simulink model "DriveSimulation"  (R2019b)
settings: Solver=FixedStepAuto  StartTime=0.0  StopTime=inf  FixedStep=dt  RelTol=1e-3
model workspace (MAT data in the model file):
  AcceNoisePower = 0.01
  AcceNoiseStd = 0.1
  AcceTs = 0.01
  ControlTs = 0.1
  DeltaNoiseStd = 0.000174532925199
  GPSNoisePower = 0.001
  GPSNoiseStd = 1
  GPSTs = 0.5
  GyroNoisePower = 0.001
  GyroNoiseStd = 0.000174532925199
  GyroTs = 0.01
  L = 2
  SteeringRange = 0.837758040957
  Ts = 0.01
  Var = 0
  Vmax = 41.6666666667
  dt = 0.01
undefined symbols (not defined in the file): DiscIntNeverNeededParam
libraries: simulink x2, robotmobilelib x1, sim3dlib x1, sim3dautolib x1, aerolibanimutils x1
settings Model: Creator=alons  LastModifiedBy=alons
settings DataIOCC: ReturnWorkspaceOutputs=off
settings DebuggingCC: ArithmeticOperatorsInVariantConditions=warning
settings SFSimCC: CustomCodeUndefinedFunction=UseInterfaceOnly

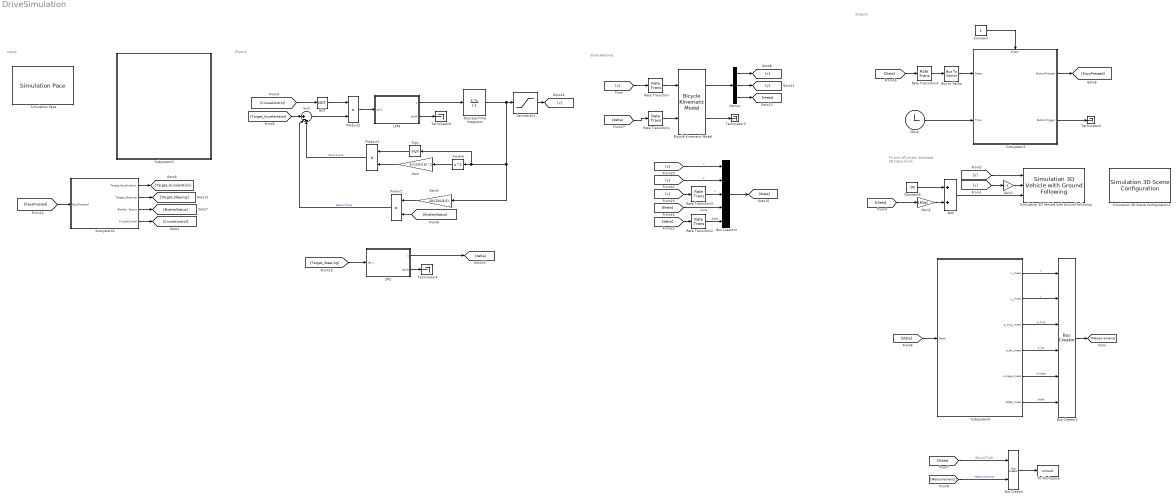
== system DriveSimulation ==
  note: Physics
  note: State Advance
  note: Inputs
  note: Outputs
  note: To turn off unreal:
      | Annotate 3D scene block
  Add : Sum
  Bicycle Kinematic Model : robotmobilelib/Bicycle Kinematic Model  VehicleInputs=Vehicle Speed & Steering Angle  WheelBase=L  VehicleSpeedRange=[-Vmax/3 Vmax]  MaxSteeringAngle=SteeringRange/2  InitialState=[0; 0; pi/2]  SimulateUsing=Interpreted execution
      settings: SourceProductName=Robotics System Toolbox  SourceProductBaseCode=RO
  Bus Creator : BusCreator  Inputs=2
  Bus Creator2 : BusCreator  Inputs=6
  Bus Creator3 : BusCreator  Inputs=5
  Bus to Vector : BusToVector
  Clock : Clock
  Constant : Constant  SampleTime=0
      settings: OpenFcn=|
      | if get_param(gcbh,'value')-48
      |    set_param(gcbh,'value','0','backgroundcolor','red');
      | else
      |    set_param(gcbh,'value','1','backgroundcolor','green');
      | end
  Constant6 : Constant  Value=-90
  Demux : Demux  Outputs=3
  Discrete-Time Integrator : DiscreteIntegrator  SampleTime=-1  ICPrevOutput=DiscIntNeverNeededParam  ICPrevScaledInput=DiscIntNeverNeededParam
  Gain : Gain  Gain=5/(150/3.6)^2
  Gain1 : Gain  Gain=-1
  Gain2 : Gain  Gain=180/pi
  Gain3 : Gain  Gain=20/(150/3.6)
  LPF2 : Subsystem  mask{Freq=2}
      mask prompts: Freq "LPF Freq [Hz]"
      mask Display: fprintf('LPF %g[Hz]',Freq);
  LPF3 : Subsystem  mask{Freq=2}
      mask prompts: Freq "LPF Freq [Hz]"
      mask Display: fprintf('LPF %g[Hz]',Freq);
  NOT : Logic  Operator=NOT  AllPortsSameDT=off  OutDataTypeStr=boolean
  Product : Product
  Product1 : Product
  Product2 : Product
  Rate Transition{,1..3} (4 alike) : RateTransition  OutPortSampleTime=dt
  Rate Transition4 : RateTransition  OutPortSampleTime=ControlTs
  Saturation1 : Saturate  UpperLimit=Vmax  LowerLimit=-Vmax/3
  Sign : Signum
  Simulation 3D Scene Configuration1 : sim3dlib/Simulation 3D Scene Configuration  Priority=0  SceneDesc=Curved road  vehTagList={'Scene Origin';'SimulinkVehicle1'}  vehTag=SimulinkVehicle1  OpVisEn=off  Ts=ControlTs  ProjectFormat=Executable  ProjectName=VehicleSimulation.exe  sensorTag=MainCamera1  sensorId=1  sensorName=MainCamera1  mountLoc=Origin  offsetFlag=off  tmountOffset=[0, 0, 0]  rmountOffset=[0, 0, 0]  HorizontalResolution=1280  VerticalResolution=720  HorizontalFOV=60  mountPoint=[0 0 0]  mountOrientation=[0 0 0]  aMode=3  ID=1
      settings: SourceProductName=Automated Driving Toolbox  SourceProductBaseCode=DR
  Simulation 3D Vehicle with Ground Following : sim3dautolib/Simulation 3D Vehicle with Ground Following  Priority=-1  PassVehMesh=Muscle car  VehColor=Red  InitialPos=[0, 0, 0]  InitialRot=[0, 0, 0]  ActorName=SimulinkVehicle1  SampleTime=-1  ActorType=SimulinkVehicle  ID=1  aMode=3  ActorTag=SimulinkVehicle1  CoordinateScheme=ISO  TransformOutportEnabled=off
      settings: SourceProductName=Automated Driving Toolbox  SourceProductBaseCode=DR
  Simulation Pace : aerolibanimutils/Simulation Pace  SimulationPace=1  SleepMode=Auto  OutputPaceError=off  SampleTime=dt
  Square : Math  Operator=square  SignedPower=off  SaturateOnIntegerOverflow=on
  Subsystem1 : Subsystem  InitFcn=|  mask{dt=0.01, ControlTs=0.1, AcceTs=0.01, GyroTs=0.01, GPSTs=0.5, AcceNoiseStd=0.1, GyroNoiseStd=0.01*pi/180, GPSNoiseStd=1, DeltaNoiseStd=0.01/180*pi, L=2, Vmax=150/3.6, SteeringRange=48/180*pi}
      | mdlWks=get_param(bdroot,'ModelWorkspace')
      | par = get_param(gcb,'DialogParameters');
      | fnames = fieldnames(par);
      | for ipar=1:length(fnames)
      |    num=str2num(get_param(gcb,fnames{ipar}));
      |    mdlWks.assignin(fnames{ipar},num);
      | end
      | 
      | clear par fnames ipar num mdlWks;
      mask prompts: dt "Physics Time Sample [s]"; ControlTs "Control Time Sample [s]"; AcceTs "Accelerometer Time Sample [s]"; GyroTs "Gyro Time Sample [s]"; GPSTs "GPS Time Sample [s]"; AcceNoiseStd "Accelerometer Noise std [m/s^2]"; GyroNoiseStd "Gyro Noise std [rad/s]"; GPSNoiseStd "GPS Noise std [m]"; DeltaNoiseStd "Steering Wheel Noise std [rad]"; L "Bicycle Length [m]"; Vmax "Maximum Velocity [m/s]"; SteeringRange "Steering Range [rad]"
      mask Display:
      | str=[
      |     'Model Workspace Parameters \n\n\n',...
      |     'Physics Sample dt = %g[s]\n\n',...
      |     'Control Sample ControlTs = %g[s]\n\n',...
      |     'Accelerometer Sample AcceTs = %g[s]\n\n',...
      |     'Gyro Sample GyroTs = %g[s]\n\n',...
      |     'GPS Sample GpsTs = %g[s]\n\n',...
      |     'Accelerometer Noise std = %g[m/s^2]\n\n',...
      |     'Gyro Noise std = %g[rad/s^2]\n\n',...
      |     'GPS Noise std = %g[m]\n\n',...
      |     'Steering Wheel Noise std = %g[m]\n\n',...
      |     'Bicycle Length L = %g[m]\n\n',...
      |     'Maximum Velocity Vmax = %g[m/s]\n\n',...
      |     'SteeringRange = %g[rad]\n\n',...
      |     ];
      | fprintf(str,dt,ControlTs,AcceTs,GyroTs,GPSTs,...
      |     AcceNoiseStd,GyroNoiseStd,GPSNoiseStd,DeltaNoiseStd,L,Vmax,SteeringRange);
  Subsystem2 : Subsystem
      settings: OpenFcn=|
      | UserData = get_param([gcb,'/AnimationSfcn'],'UserData');
      | Fig = UserData.Figure;
      | if ishghandle(Fig,'figure');
      |    %bring to the front:
      |    figure(Fig);
      | end
      mask Display:
      | t=linspace(0,2*pi,20);
      | plot(cos(t),sin(t));
      | 
      | x=[-0.4,-0.4,0.6,-0.4];
      | y=[-0.5,0.5,0,-0.5];
      | plot(x,y)
      | 
      | disp('Drive Simulator')
  Subsystem3 : Subsystem
  Subsystem4 : Subsystem
      mask Display: disp('Sensor Readings')
  Sum : Sum  Inputs=||+--
  Terminator{2..5} (4 alike) : Terminator
  To Workspace : ToWorkspace  VariableName=simout  SaveFormat=Timeseries  SampleTime=-1
  wires:
  Constant/1 -> Subsystem2/Enable
  Clock/1 -> Subsystem2/2(Time)
  Subsystem3/1(Target_Acceleration) -> [Target_Acceleration]
  Subsystem3/2(Target_Steering) -> [Target_Steering]
  Bus to Vector/1 -> Subsystem2/1(State)
  Subsystem2/1(ButtonPressed) -> [KeysPressed]
  Subsystem2/2(ButtonTrigger) -> Terminator2/1
  Subsystem4/5(omega_meas) -> Bus Creator2/5  "omega"
  Subsystem4/4(a_lat_meas) -> Bus Creator2/4  "a_lat"
  Subsystem4/3(a_long_meas) -> Bus Creator2/3  "a_long"
  Subsystem4/2(y_meas) -> Bus Creator2/2  "y"
  Subsystem4/1(x_meas) -> Bus Creator2/1  "x"
  Subsystem4/6(delta_meas) -> Bus Creator2/6  "delta"
  [KeysPressed] -> Subsystem3/1(KeysPressed)
  Bicycle Kinematic Model/2 -> Terminator3/1
  Bicycle Kinematic Model/1 -> Demux/1
  Demux/1 -> [x]
  Demux/2 -> [y]
  Demux/3 -> [theta]
  [x] -> Bus Creator3/1  "x"
  [y] -> Bus Creator3/2  "y"
  [v] -> Rate Transition3/1
  [theta] -> Bus Creator3/4  "theta"
  [delta] -> Rate Transition2/1
  Bus Creator3/1 -> [State]
  [State] -> Rate Transition4/1
  [Target_Steering] -> LPF2/1(ref s)
  LPF2/1(s) -> [delta]
  LPF2/2(ds/dt) -> Terminator4/1
  [delta] -> Rate Transition1/1
  [v] -> Rate Transition/1
  [State] -> Subsystem4/1(State)
  LPF3/1(s) -> Discrete-Time Integrator/1
  LPF3/2(ds/dt) -> Terminator5/1
  [Target_Acceleration] -> Sum/1
  Square/1 -> Gain/1
  Discrete-Time Integrator/1 -> Gain3/1, Sign/1, Square/1, Saturation1/1
  Subsystem3/3(Brakes  Status) -> [BrakesStatus]
  Gain3/1 -> Product/1
  Product/1 -> Sum/2  "Brake Force"
  [BrakesStatus] -> Product/2
  [theta] -> Gain2/1
  [y] -> Simulation 3D Vehicle with Ground Following/1
  Constant6/1 -> Add/1
  Gain2/1 -> Add/2
  Add/1 -> Simulation 3D Vehicle with Ground Following/3
  [x] -> Gain1/1
  Gain1/1 -> Simulation 3D Vehicle with Ground Following/2
  Product1/1 -> Sum/3  "Wind Force"
  Gain/1 -> Product1/2
  Sign/1 -> Product1/1
  Bus Creator2/1 -> [Measurements]
  Bus Creator/1 -> To Workspace/1
  [State] -> Bus Creator/1  "Ground Truth"
  [Measurements] -> Bus Creator/2  "Measurements"
  Subsystem3/4(CruiseControl) -> [CruiseControl]
  Sum/1 -> Product2/2
  [CruiseControl] -> NOT/1
  NOT/1 -> Product2/1
  Product2/1 -> LPF3/1(ref s)
  Saturation1/1 -> [v]
  Rate Transition/1 -> Bicycle Kinematic Model/1
  Rate Transition1/1 -> Bicycle Kinematic Model/2
  Rate Transition2/1 -> Bus Creator3/5  "delta"
  Rate Transition3/1 -> Bus Creator3/3  "v"
  Rate Transition4/1 -> Bus to Vector/1

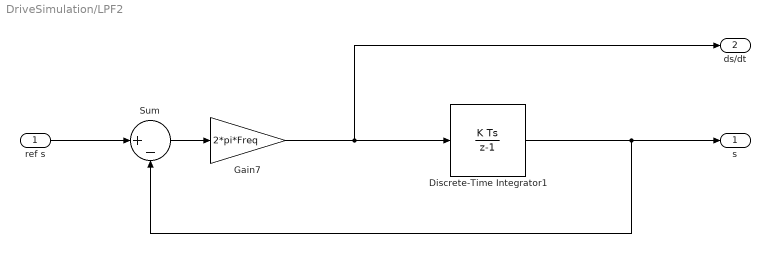
== system DriveSimulation/LPF2 ==
  ref s : Inport
  Discrete-Time Integrator1 : DiscreteIntegrator  SampleTime=-1  ICPrevOutput=DiscIntNeverNeededParam  ICPrevScaledInput=DiscIntNeverNeededParam
  Gain7 : Gain  Gain=2*pi*Freq
  Sum : Sum  Inputs=|+-
  s : Outport  VectorParamsAs1DForOutWhenUnconnected=off
  ds/dt : Outport  Port=2  VectorParamsAs1DForOutWhenUnconnected=off
  wires:
  Discrete-Time Integrator1/1 -> Sum/2, s/1
  Sum/1 -> Gain7/1
  ref s/1 -> Sum/1
  Gain7/1 -> Discrete-Time Integrator1/1, ds/dt/1

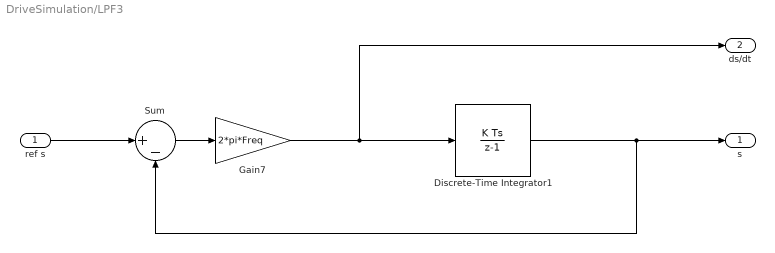
== system DriveSimulation/LPF3 ==
  ref s : Inport
  Discrete-Time Integrator1 : DiscreteIntegrator  SampleTime=-1  ICPrevOutput=DiscIntNeverNeededParam  ICPrevScaledInput=DiscIntNeverNeededParam
  Gain7 : Gain  Gain=2*pi*Freq
  Sum : Sum  Inputs=|+-
  s : Outport  VectorParamsAs1DForOutWhenUnconnected=off
  ds/dt : Outport  Port=2  VectorParamsAs1DForOutWhenUnconnected=off
  wires:
  Discrete-Time Integrator1/1 -> Sum/2, s/1
  Sum/1 -> Gain7/1
  ref s/1 -> Sum/1
  Gain7/1 -> Discrete-Time Integrator1/1, ds/dt/1

== system DriveSimulation/Subsystem1 ==

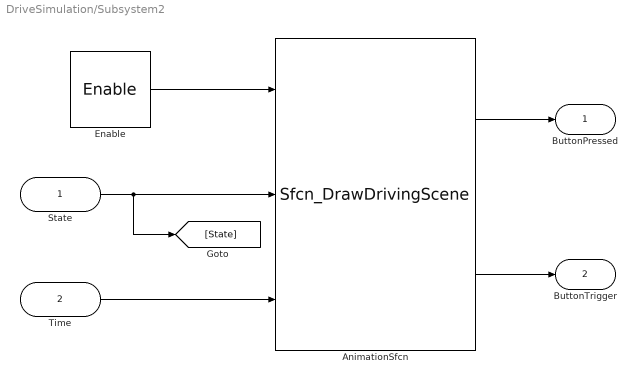
== system DriveSimulation/Subsystem2 ==
  State : Inport
  Time : Inport  Port=2
  Enable : EnablePort  StatesWhenEnabling=reset  ShowOutputPort=on
  AnimationSfcn : M-S-Function  FunctionName=Sfcn_DrawDrivingScene  Parameters=ControlTs,L,Vmax
  ButtonPressed : Outport  VectorParamsAs1DForOutWhenUnconnected=off
  ButtonTrigger : Outport  Port=2  VectorParamsAs1DForOutWhenUnconnected=off
  wires:
  Enable/1 -> AnimationSfcn/1
  AnimationSfcn/1 -> ButtonPressed/1
  AnimationSfcn/2 -> ButtonTrigger/1
  Time/1 -> AnimationSfcn/3
  State/1 -> [State], AnimationSfcn/2

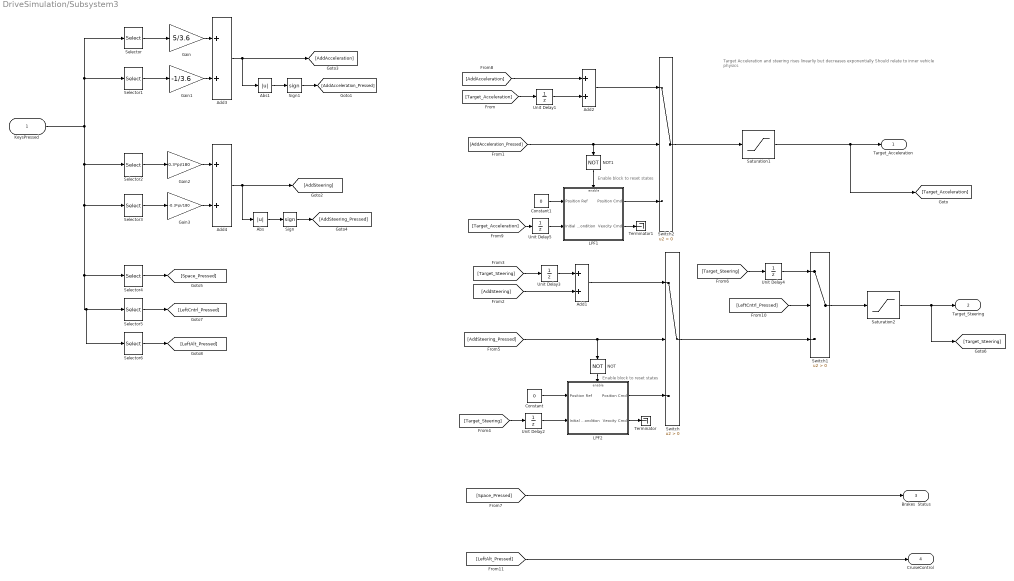
== system DriveSimulation/Subsystem3 ==
  note: Enable block to reset states
  note: Enable block to reset states
  note: Target Acceleration and steering rises linearliy but decreases exponentially
      | Should relate to inner vehicle physics
  KeysPressed : Inport
  Abs : Abs
  Abs1 : Abs
  Add{1..4} (4 alike) : Sum
  Constant : Constant  Value=0
  Constant1 : Constant  Value=0
  Gain : Gain  Gain=5/3.6
  Gain1 : Gain  Gain=-1/3.6
  Gain2 : Gain  Gain=0.3*pi/180
  Gain3 : Gain  Gain=-0.3*pi/180
  LPF1 : Subsystem  mask{PosBW=1, Vel_Max=inf, Vel_Min=-inf}
      mask prompts: PosBW "Position BW [Hz]"; Vel_Max "Maximum Velocity"; Vel_Min "Minimum Velocity"
      mask Display: fprintf('Resetable LPF %.3g[Hz] \n/w Vel Limits',PosBW);
  LPF2 : Subsystem  mask{PosBW=0.5, Vel_Max=inf, Vel_Min=-inf}
      mask prompts: PosBW "Position BW [Hz]"; Vel_Max "Maximum Velocity"; Vel_Min "Minimum Velocity"
      mask Display: fprintf('Resetable LPF %.3g[Hz] \n/w Vel Limits',PosBW);
  NOT : Logic  Operator=NOT  AllPortsSameDT=off  OutDataTypeStr=boolean
  NOT1 : Logic  Operator=NOT  AllPortsSameDT=off  OutDataTypeStr=boolean
  Saturation1 : Saturate  UpperLimit=10  LowerLimit=-10
  Saturation2 : Saturate  UpperLimit=SteeringRange/2  LowerLimit=-SteeringRange/2
  Selector : Selector  InputPortWidth=7  IndexOptions=Index vector (dialog)  Indices=1  OutputSizes=1
  Selector1 : Selector  InputPortWidth=7  IndexOptions=Index vector (dialog)  Indices=2  OutputSizes=1
  Selector2 : Selector  InputPortWidth=7  IndexOptions=Index vector (dialog)  Indices=3  OutputSizes=1
  Selector3 : Selector  InputPortWidth=7  IndexOptions=Index vector (dialog)  Indices=4  OutputSizes=1
  Selector4 : Selector  InputPortWidth=7  IndexOptions=Index vector (dialog)  Indices=5  OutputSizes=1
  Selector5 : Selector  InputPortWidth=7  IndexOptions=Index vector (dialog)  Indices=6  OutputSizes=1
  Selector6 : Selector  InputPortWidth=7  IndexOptions=Index vector (dialog)  Indices=7  OutputSizes=1
  Sign : Signum
  Sign1 : Signum
  Switch : Switch  Criteria=u2 > Threshold
  Switch1 : Switch  Criteria=u2 > Threshold
  Switch2 : Switch  Criteria=u2 > Threshold
  Terminator : Terminator
  Terminator1 : Terminator
  Unit Delay{1..5} (5 alike) : UnitDelay  SampleTime=-1  HasFrameUpgradeWarning=on
  Target_Acceleration : Outport  VectorParamsAs1DForOutWhenUnconnected=off
  Target_Steering : Outport  Port=2  VectorParamsAs1DForOutWhenUnconnected=off
  Brakes  Status : Outport  Port=3  VectorParamsAs1DForOutWhenUnconnected=off
  CruiseControl : Outport  Port=4  VectorParamsAs1DForOutWhenUnconnected=off
  wires:
  [Target_Acceleration] -> Unit Delay1/1
  Unit Delay1/1 -> Add2/2
  Add2/1 -> Switch2/1
  [AddAcceleration] -> Add2/1
  Add4/1 -> Abs/1, [AddSteering]
  Selector/1 -> Gain/1
  Selector1/1 -> Gain1/1
  Gain1/1 -> Add3/2
  Gain/1 -> Add3/1
  Add3/1 -> Abs1/1, [AddAcceleration]
  Selector2/1 -> Gain2/1
  Selector3/1 -> Gain3/1
  Gain2/1 -> Add4/1
  Gain3/1 -> Add4/2
  Switch2/1 -> Saturation1/1
  KeysPressed/1 -> Selector6/1, Selector5/1, Selector4/1, Selector3/1, Selector2/1, Selector/1, Selector1/1
  Abs/1 -> Sign/1
  Sign/1 -> [AddSteering_Pressed]
  Selector4/1 -> [Space_Pressed]
  Switch1/1 -> Saturation2/1
  Unit Delay2/1 -> LPF2/2(Initial Condition)
  [Target_Steering] -> Unit Delay3/1
  [Target_Steering] -> Unit Delay2/1
  LPF2/2(Veocity Cmd) -> Terminator/1
  Unit Delay3/1 -> Add1/1
  [AddSteering] -> Add1/2
  LPF2/1(Position Cmd) -> Switch/3
  Constant/1 -> LPF2/1(Position Ref)
  NOT/1 -> LPF2/Enable
  [AddSteering_Pressed] -> NOT/1, Switch/2
  Add1/1 -> Switch/1
  [LeftCntrl_Pressed] -> Switch1/2
  [Target_Steering] -> Unit Delay4/1
  Unit Delay4/1 -> Switch1/1
  Switch/1 -> Switch1/3
  Abs1/1 -> Sign1/1
  Sign1/1 -> [AddAcceleration_Pressed]
  Unit Delay5/1 -> LPF1/2(Initial Condition)
  LPF1/1(Position Cmd) -> Switch2/3
  LPF1/2(Veocity Cmd) -> Terminator1/1
  Constant1/1 -> LPF1/1(Position Ref)
  [AddAcceleration_Pressed] -> Switch2/2, NOT1/1
  NOT1/1 -> LPF1/Enable
  [Target_Acceleration] -> Unit Delay5/1
  Saturation1/1 -> Target_Acceleration/1, [Target_Acceleration]
  Saturation2/1 -> [Target_Steering], Target_Steering/1
  Selector5/1 -> [LeftCntrl_Pressed]
  [Space_Pressed] -> Brakes  Status/1
  Selector6/1 -> [LeftAlt_Pressed]
  [LeftAlt_Pressed] -> CruiseControl/1

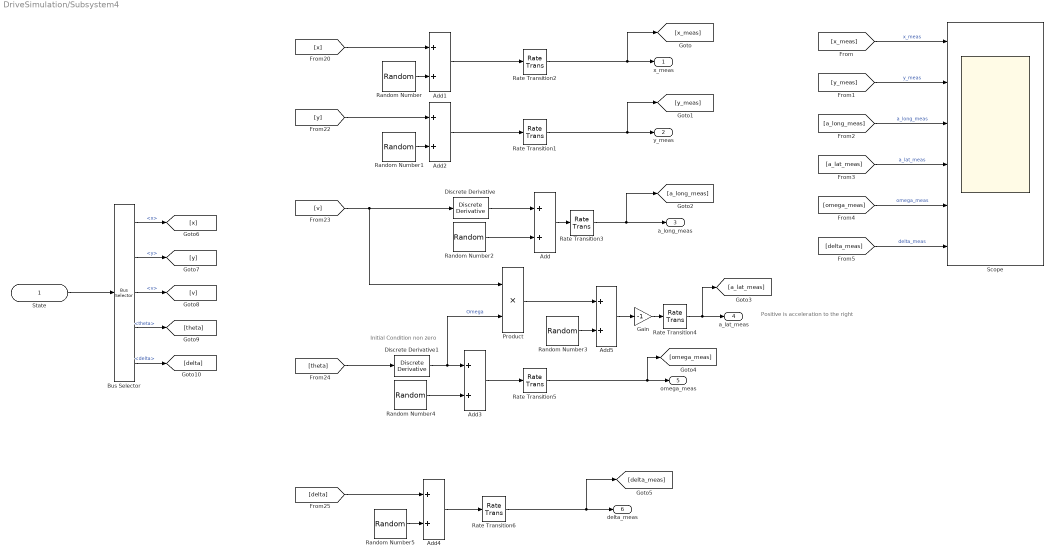
== system DriveSimulation/Subsystem4 ==
  note: Initial Condition non zero
  note: Positive is acceleration to the right
  State : Inport
  Add{,1..5} (6 alike) : Sum
  Bus Selector : BusSelector  OutputSignals=x,y,v,theta,delta
  Discrete Derivative : simulink/Discrete/Discrete Derivative  gainval=1.0  ICPrevScaledInput=0.0  OutMin=[]  OutMax=[]  OutDataType=fixdt(1, 16)  OutScaling=2^-10  DoSatur=off
  Discrete Derivative1 : simulink/Discrete/Discrete Derivative  gainval=1.0  ICPrevScaledInput=pi/2/dt  OutMin=[]  OutMax=[]  OutDataType=fixdt(1, 16)  OutScaling=2^-10  DoSatur=off
  Gain : Gain  Gain=-1
  Product : Product
  Random Number : RandomNumber  Variance=(GPSNoiseStd^2)
  Random Number1 : RandomNumber  Variance=(GPSNoiseStd^2)  Seed=2
  Random Number2 : RandomNumber  Variance=AcceNoiseStd^2  Seed=3
  Random Number3 : RandomNumber  Variance=AcceNoiseStd^2  Seed=4
  Random Number4 : RandomNumber  Variance=GyroNoiseStd  Seed=5
  Random Number5 : RandomNumber  Variance=(DeltaNoiseStd^2)  Seed=2
  Rate Transition1 : RateTransition  OutPortSampleTime=GPSTs
  Rate Transition2 : RateTransition  OutPortSampleTime=GPSTs
  Rate Transition3 : RateTransition  OutPortSampleTime=AcceTs
  Rate Transition4 : RateTransition  OutPortSampleTime=AcceTs
  Rate Transition5 : RateTransition  OutPortSampleTime=GyroTs
  Rate Transition6 : RateTransition  OutPortSampleTime=GPSTs
  Scope : Scope  NumInputPorts=6
  x_meas : Outport  VectorParamsAs1DForOutWhenUnconnected=off
  y_meas : Outport  Port=2  VectorParamsAs1DForOutWhenUnconnected=off
  a_long_meas : Outport  Port=3  VectorParamsAs1DForOutWhenUnconnected=off
  a_lat_meas : Outport  Port=4  VectorParamsAs1DForOutWhenUnconnected=off
  omega_meas : Outport  Port=5  VectorParamsAs1DForOutWhenUnconnected=off
  delta_meas : Outport  Port=6  VectorParamsAs1DForOutWhenUnconnected=off
  wires:
  Random Number/1 -> Add1/2
  Random Number2/1 -> Add/2
  Random Number3/1 -> Add5/2
  Random Number1/1 -> Add2/2
  [v] -> Product/1, Discrete Derivative/1
  Discrete Derivative1/1 -> Product/2, Add3/1  "Omega"
  Product/1 -> Add5/1
  [y] -> Add2/1
  Random Number4/1 -> Add3/2
  Add1/1 -> Rate Transition2/1
  Add/1 -> Rate Transition3/1
  Add3/1 -> Rate Transition5/1
  Add2/1 -> Rate Transition1/1
  [x] -> Add1/1
  Add5/1 -> Gain/1
  [theta] -> Discrete Derivative1/1
  Gain/1 -> Rate Transition4/1
  [x_meas] -> Scope/1  "x_meas"
  [y_meas] -> Scope/2  "y_meas"
  [a_long_meas] -> Scope/3  "a_long_meas"
  [a_lat_meas] -> Scope/4  "a_lat_meas"
  [omega_meas] -> Scope/5  "omega_meas"
  Rate Transition2/1 -> [x_meas], x_meas/1
  Rate Transition1/1 -> [y_meas], y_meas/1
  Rate Transition3/1 -> [a_long_meas], a_long_meas/1
  Rate Transition4/1 -> [a_lat_meas], a_lat_meas/1
  Rate Transition5/1 -> [omega_meas], omega_meas/1
  Discrete Derivative/1 -> Add/1
  [delta] -> Add4/1
  Rate Transition6/1 -> [delta_meas], delta_meas/1
  Add4/1 -> Rate Transition6/1
  Random Number5/1 -> Add4/2
  [delta_meas] -> Scope/6  "delta_meas"
  State/1 -> Bus Selector/1
  Bus Selector/1 -> [x]  "<x>"
  Bus Selector/2 -> [y]  "<y>"
  Bus Selector/3 -> [v]  "<v>"
  Bus Selector/4 -> [theta]  "<theta>"
  Bus Selector/5 -> [delta]  "<delta>"

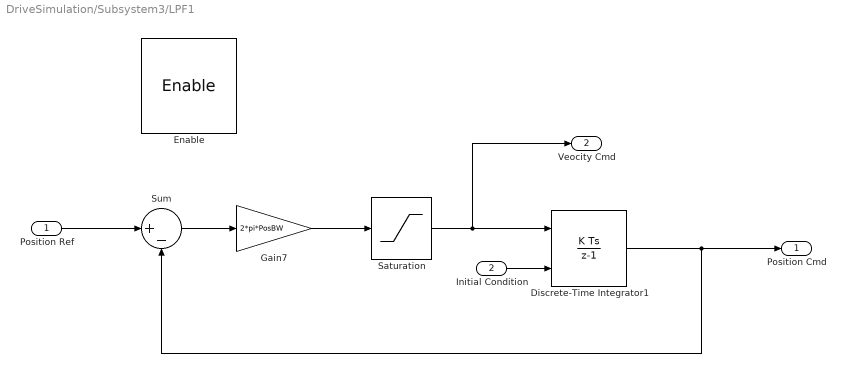
== system DriveSimulation/Subsystem3/LPF1 ==
  Position Ref : Inport
  Initial Condition : Inport  Port=2
  Enable : EnablePort  StatesWhenEnabling=reset
  Discrete-Time Integrator1 : DiscreteIntegrator  InitialConditionSource=external  SampleTime=-1  ICPrevOutput=DiscIntNeverNeededParam  ICPrevScaledInput=DiscIntNeverNeededParam
  Gain7 : Gain  Gain=2*pi*PosBW
  Saturation : Saturate  UpperLimit=Vel_Max  LowerLimit=Vel_Min
  Sum : Sum  Inputs=|+-
  Position Cmd : Outport  VectorParamsAs1DForOutWhenUnconnected=off
  Veocity Cmd : Outport  Port=2  VectorParamsAs1DForOutWhenUnconnected=off
  wires:
  Position Ref/1 -> Sum/1
  Sum/1 -> Gain7/1
  Gain7/1 -> Saturation/1
  Discrete-Time Integrator1/1 -> Position Cmd/1, Sum/2
  Saturation/1 -> Veocity Cmd/1, Discrete-Time Integrator1/1
  Initial Condition/1 -> Discrete-Time Integrator1/2

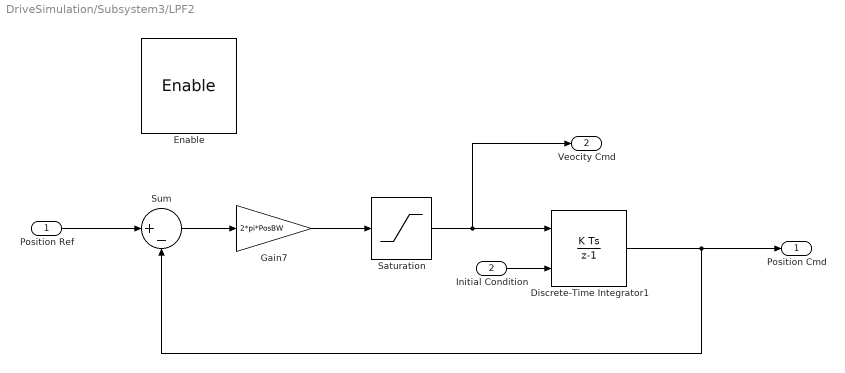
== system DriveSimulation/Subsystem3/LPF2 ==
  Position Ref : Inport
  Initial Condition : Inport  Port=2
  Enable : EnablePort  StatesWhenEnabling=reset
  Discrete-Time Integrator1 : DiscreteIntegrator  InitialConditionSource=external  SampleTime=-1  ICPrevOutput=DiscIntNeverNeededParam  ICPrevScaledInput=DiscIntNeverNeededParam
  Gain7 : Gain  Gain=2*pi*PosBW
  Saturation : Saturate  UpperLimit=Vel_Max  LowerLimit=Vel_Min
  Sum : Sum  Inputs=|+-
  Position Cmd : Outport  VectorParamsAs1DForOutWhenUnconnected=off
  Veocity Cmd : Outport  Port=2  VectorParamsAs1DForOutWhenUnconnected=off
  wires:
  Position Ref/1 -> Sum/1
  Sum/1 -> Gain7/1
  Gain7/1 -> Saturation/1
  Discrete-Time Integrator1/1 -> Position Cmd/1, Sum/2
  Saturation/1 -> Veocity Cmd/1, Discrete-Time Integrator1/1
  Initial Condition/1 -> Discrete-Time Integrator1/2
